simulink model "Boeing787_NewMission_ElectricalThermal"  (R2016a)
settings: Solver=ode23tb  SolverMode=SingleTasking  StartTime=0.0  StopTime=18000  RelTol=1e-3
InitFcn:
  | load('SampleOutput.mat')
  | 
  | load('SampleFuelBurn.mat')
StartFcn:
  | tic
StopFcn:
  | ttt = toc
  | tend = eval(get_param(bdroot,'StopTime'));
  | disp(['Total Simulation Time (s) = ' num2str(ttt) 's']);
  | RTR =  ttt/tend
  | disp(['Simulation Speed is ' num2str(tend/ttt) 'x faster than real-time']);
undefined symbols (not defined in the file): CurrentMission, FuelBurn, seed
libraries: PowerFlowLib x18, simulink x12, powerlib_meascontrol x1
(part 17 of 17)

== matlab function Boeing787_NewMission_ElectricalThermal/Electrical/Thermal Interface/Battery Thermal Model/MATLAB Function ==
  data: Ploss input; Tdot output; Tf input; Ta input; mdot_f input; Tgen input
function Tdot = Battery_loss(Ploss, Tf, Ta, mdot_f, Tgen)
%% Constants

% generator parameters
Cp_gen  = 0.49*1000;                     % Cp of carbon steel [J/kg-K]
m_gen   = 250;                        % mass of generator [kg]
L_gen   = 0.5;                        % length of generator [m]
D_gen   = 0.3;                        % diameter of generator [m]

% fuel parameters
nu_f    = 4.77*10^-6;                    % kinematic viscosity of JP8 [m^2/s]
k_f     = 0.115;                         % thermal conductivity of JP8[W/m-K]
rho_f   = 900;                           % density [kg/m^3]
Cp_f    = 1900;                          % Cp of Jp8 [J/kg-K]

% air parameters
nu_a    = 1.568*10^-5;                   % kinematic viscosity of air [m^2/s]
k_a     = 0.0257;                        % thermal conductivity of air[W/m-K]
rho_a   = 1.205;                         % density [kg/m^3]
Cp_a    = 1005;                          % Cp of Jp8 [J/kg-K]


% outer surface area of generator
A_a   = pi*D_gen*L_gen + 2*pi/4*D_gen^2;

% assume the inner surface area for the water jacket is a series of tubes
nTubes = 15;                        % number of tubes
D_tubes = .02;                      % diameter of tubes [m]

A_f   = nTubes*(pi*D_tubes*L_gen);  % surface area of fuel interactions

%% Calculations
% fuel
V_f = mdot_f / rho_f / (D_tubes^2/4*pi); 

Pr_f = rho_f * nu_f * Cp_f / k_f;
Re_f = V_f * L_gen / nu_f;

h_f = 0.037 * Re_f^(4/5) * Pr_f^(1/3) * k_f / L_gen;

% air
V_a = 3; % assume free stream velocity is 3m/s

Pr_a = rho_a * nu_a * Cp_a / k_a;
Re_a = V_a * L_gen / nu_a;

h_a = 0.037 * Re_a^(4/5) * Pr_a^(1/3) * k_a / L_gen;




Tdot = 1/(m_gen*Cp_gen) * ( Ploss + (Tf - Tgen)*h_f*A_f + (Ta - Tgen)*h_a*A_a);

== matlab function Boeing787_NewMission_ElectricalThermal/Electrical/Thermal Interface/Load Thermal Model/MATLAB Function ==
  data: Ploss input; Tdot output; Tf input; Ta input; mdot_f input; Tgen input
function Tdot = Generator_loss(Ploss, Tf, Ta, mdot_f, Tgen)
%% Constants

% generator parameters
Cp_gen  = 0.49*1000;                     % Cp of carbon steel [J/kg-K]
m_gen   = 250;                        % mass of generator [kg]
L_gen   = 0.5;                        % length of generator [m]
D_gen   = 0.3;                        % diameter of generator [m]

% fuel parameters
nu_f    = 4.77*10^-6;                    % kinematic viscosity of JP8 [m^2/s]
k_f     = 0.115;                         % thermal conductivity of JP8[W/m-K]
rho_f   = 900;                           % density [kg/m^3]
Cp_f    = 1900;                          % Cp of Jp8 [J/kg-K]

% air parameters
nu_a    = 1.568*10^-5;                   % kinematic viscosity of air [m^2/s]
k_a     = 0.0257;                        % thermal conductivity of air[W/m-K]
rho_a   = 1.205;                         % density [kg/m^3]
Cp_a    = 1005;                          % Cp of Jp8 [J/kg-K]


% outer surface area of generator
A_a   = pi*D_gen*L_gen + 2*pi/4*D_gen^2;

% assume the inner surface area for the water jacket is a series of tubes
nTubes = 15;                        % number of tubes
D_tubes = .02;                      % diameter of tubes [m]

A_f   = nTubes*(pi*D_tubes*L_gen);  % surface area of fuel interactions

%% Calculations
% fuel
V_f = mdot_f / rho_f / (D_tubes^2/4*pi); 

Pr_f = rho_f * nu_f * Cp_f / k_f;
Re_f = V_f * L_gen / nu_f;

h_f = 0.037 * Re_f^(4/5) * Pr_f^(1/3) * k_f / L_gen;

% air
V_a = 3; % assume free stream velocity is 3m/s

Pr_a = rho_a * nu_a * Cp_a / k_a;
Re_a = V_a * L_gen / nu_a;

h_a = 0.037 * Re_a^(4/5) * Pr_a^(1/3) * k_a / L_gen;




Tdot = 1/(m_gen*Cp_gen) * ( Ploss + (Tf - Tgen)*h_f*A_f + (Ta - Tgen)*h_a*A_a);
